simulink model "VariableFixedSteps"  (R2019b)
settings: Solver=VariableStepAuto  StartTime=0.0  StopTime=5.0  FixedStep=0.05  RelTol=1e-3
settings Model: Creator=jorge  LastModifiedBy=jorge

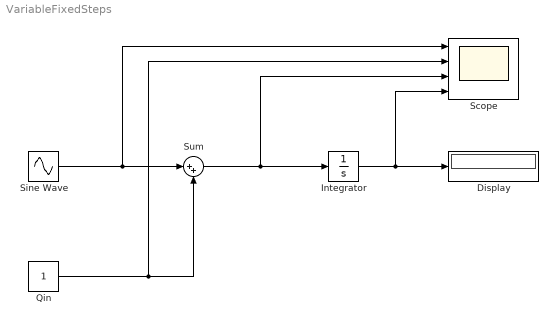
== system VariableFixedSteps ==
  Display : Display
  Integrator : Integrator
  Qin : Constant
  Scope : Scope  NumInputPorts=4
  Sine Wave : Sin  Frequency=2*pi  SampleTime=0
  Sum : Sum  Inputs=|++
  wires:
  Sine Wave/1 -> Scope/1, Sum/1
  Sum/1 -> Scope/3, Integrator/1
  Integrator/1 -> Scope/4, Display/1
  Qin/1 -> Scope/2, Sum/2
